simulink model "Final2020feb"  (R2016a)
settings: Solver=VariableStepAuto  StartTime=0.0  StopTime=10.0  RelTol=1e-3
values from neighbouring files (symbols this model uses):
  A1 = -A(1,1)    [FInal2019.m]    (also in FInal_3_12_2021.m; Final2017.m; Final2018.m; Final2020feb.m)
  A2 = -A(1,2)    [FInal2019.m]    (also in FInal_3_12_2021.m; Final2017.m; Final2018.m; Final2020feb.m)
  A3 = -A(1,3)    [FInal2019.m]    (also in FInal_3_12_2021.m; Final2017.m; Final2018.m; Final2020feb.m)
  K1 = K(1,1)    [FInal2019.m]    (also in FInal_3_12_2021.m = khat(1,1); Final2017.m; Final2018.m; Final2020feb.m = khat(1,1))
  K2 = K(1,2)    [FInal2019.m]    (also in FInal_3_12_2021.m = khat(1,2); Final2017.m; Final2018.m; Final2020feb.m = khat(1,2))
  K3 = K(1,3)    [FInal2019.m]    (also in FInal_3_12_2021.m = khat(1,3); Final2017.m; Final2018.m; Final2020feb.m = khat(1,3))
  Ki = -khat(1,4)    [FInal_3_12_2021.m]    (also in Final2020feb.m)
settings Model: Creator=alber  LastModifiedBy=alber

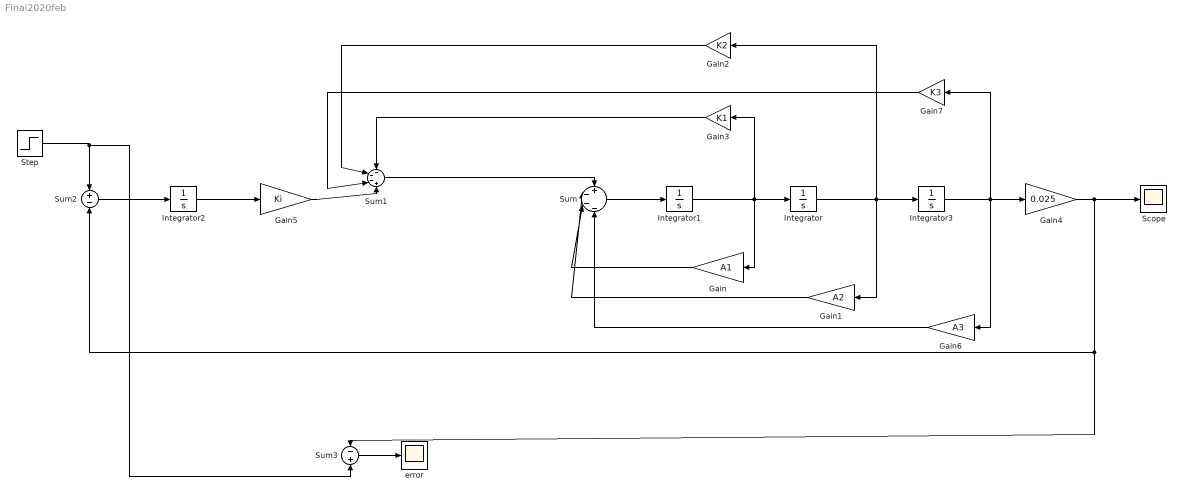
== system Final2020feb ==
  Gain : Gain  Gain=A1
  Gain1 : Gain  Gain=A2
  Gain2 : Gain  Gain=K2
  Gain3 : Gain  Gain=K1
  Gain4 : Gain  Gain=0.025
  Gain5 : Gain  Gain=Ki
  Gain6 : Gain  Gain=A3
  Gain7 : Gain  Gain=K3
  Integrator{,1..3} (4 alike) : Integrator
  Scope : Scope
  Step : Step  SampleTime=0
  Sum : Sum  Inputs=+---
  Sum1 : Sum  Inputs=---+
  Sum2 : Sum  Inputs=+-
  Sum3 : Sum  Inputs=-+
  error : Scope
  wires:
  Integrator1/1 -> Gain3/1, Gain/1, Integrator/1
  Sum/1 -> Integrator1/1
  Gain/1 -> Sum/3
  Gain1/1 -> Sum/2
  Gain3/1 -> Sum1/1
  Step/1 -> Sum3/2, Sum2/1
  Sum3/1 -> error/1
  Integrator2/1 -> Gain5/1
  Sum2/1 -> Integrator2/1
  Gain2/1 -> Sum1/2
  Sum1/1 -> Sum/1
  Gain4/1 -> Sum2/2, Sum3/1, Scope/1
  Integrator3/1 -> Gain7/1, Gain6/1, Gain4/1
  Integrator/1 -> Integrator3/1, Gain2/1, Gain1/1
  Gain5/1 -> Sum1/4
  Gain7/1 -> Sum1/3
  Gain6/1 -> Sum/4
